simulink model "LandL"  (R2018a)
settings: Solver=VariableStepAuto  StartTime=0.0  StopTime=100  FixedStep=0.0001  MaxStep=1e-2  RelTol=1e-3  EnableMultiTasking=on
values from neighbouring files (symbols this model uses):
  C = (y_hat-y_ref)'*(y_hat-y_ref)/length(y_hat)    [QELandL.m]    (also in QEPID.m)
  ks = K(4)    [QELandL.m]    (also in final_cube_alg.m = x(4))
  pi1 = K(2)*1i    [QELandL.m]    (also in final_cube_alg.m = x(2)*1i)
  pr1 = K(1)    [QELandL.m]    (also in final_cube_alg.m = x(1))
  zr = K(3)    [QELandL.m]    (also in final_cube_alg.m = x(3))
undefined symbols (not defined in the file or in its folder): A, B
libraries: simulink x3, slident x2, cstblocks x1
settings Model: Creator=rromano  LastModifiedBy=Marcelo
settings SolverCC: ZeroCrossAlgorithm=Adaptive  AutoInsertRateTranBlk=on
settings DataIOCC: LimitDataPoints=on  SaveFormat=Array  SignalLoggingSaveFormat=ModelDataLogs
settings OptimizationCC: ExpressionDepthLimit=2147483647  LifeSpan=inf
settings DebuggingCC: AlgebraicLoopMsg=none  UnderspecifiedInitializationDetection=Classic  MergeDetectMultiDrivingBlocksExec=none  MaxConsecutiveZCsMsg=none  SolverPrmCheckMsg=warning  FcnCallInpInsideContextMsg=warning  StateNameClashWarn=warning  SFUnexpectedBacktrackingDiag=warning  SFNoUnconditionalDefaultTransitionDiag=warning  SFExecutionAtInitializationDiag=none
settings HardwareCC: ProdBitPerPointer=32  ProdBitPerSizeT=32  ProdBitPerPtrDiffT=32  ProdLargestAtomicFloat=None  ProdIntDivRoundTo=Undefined  ProdEndianess=Unspecified  ProdWordSize=32  ProdHWDeviceType=32-bit Generic
settings ModelReferenceCC: PropagateSignalLabelsOutOfModel=off
settings CodeAppCC: StateflowObjectComments=on
settings GRTTargetCC: TargetLangStandard=C89/C90 (ANSI)  GeneratePreprocessorConditionals=Disable all  CombineOutputUpdateFcns=off  GRTInterface=on
settings ConfigComp: CovMetricSettings=dw  CovHtmlReporting=on  CovSaveCumulativeToWorkspaceVar=on  CovSaveSingleToWorkspaceVar=on  CovExternalEMLEnable=off

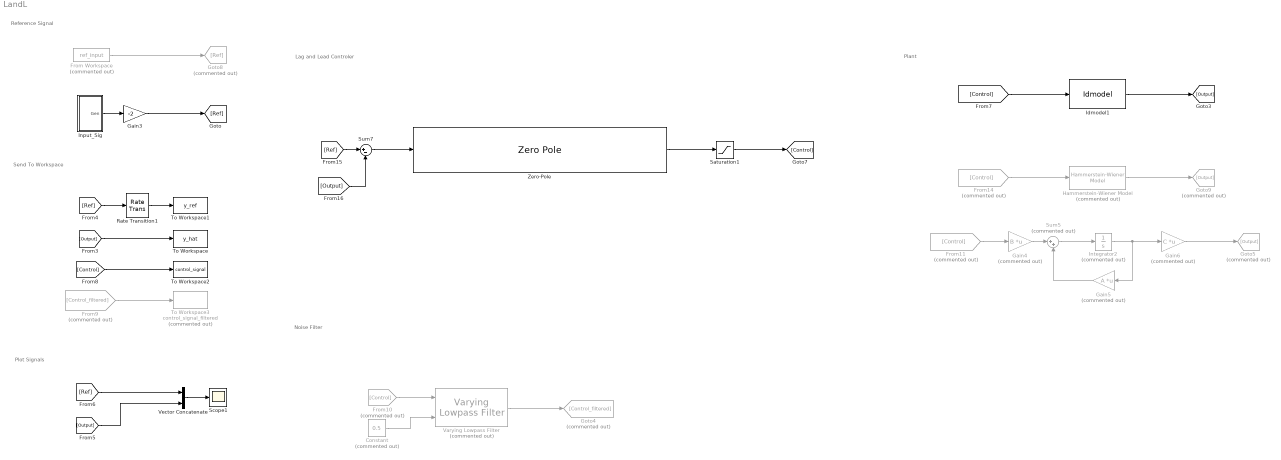
== system LandL ==
  note: Noise Filter
  note: Plot Signals
  note: Send To Workspace
  note: Reference Signal
  note: Lag and Lead Controler
  note: Plant
  Constant : Constant  Commented=on  Value=0.5
  From Workspace : FromWorkspace  Commented=on  VariableName=ref_input  SampleTime=0
  From10 : From  Commented=on  GotoTag=Control
  From11 : From  Commented=on  GotoTag=Control
  From14 : From  Commented=on  GotoTag=Control
  From9 : From  Commented=on  GotoTag=Control_filtered
  Gain3 : Gain  Gain=-2
  Gain4 : Gain  Commented=on  Gain=B  Multiplication=Matrix(K*u)
  Gain5 : Gain  Commented=on  Gain=A  Multiplication=Matrix(K*u)
  Gain6 : Gain  Commented=on  Gain=C  Multiplication=Matrix(K*u)
  Goto4 : Goto  Commented=on  GotoTag=Control_filtered
  Goto5 : Goto  Commented=on  GotoTag=Output
  Goto8 : Goto  Commented=on  GotoTag=Ref
  Goto9 : Goto  Commented=on  GotoTag=Output
  Hammerstein-Wiener Model : slident/Models/Hammerstein-Wiener Model  Commented=on  sys=linear_app  IC=Zero  X0i=0
      settings: SourceProductName=System Identification Toolbox  SourceProductBaseCode=ID
  Idmodel1 : slident/Models/Idmodel  sys=linear_app  IC=0  noi=off  seed=[]
      settings: SourceProductName=System Identification Toolbox  SourceProductBaseCode=ID
  Input_Sig : Subsystem
  Integrator2 : Integrator  Commented=on  ZeroCross=off
  Rate Transition1 : RateTransition  OutPortSampleTime=0.2
  Saturation1 : Saturate  UpperLimit=5000  LowerLimit=-5000
  Scope1 : Scope
  Sum5 : Sum  Commented=on  Inputs=|++
  Sum7 : Sum  Inputs=|+-
  To Workspace : ToWorkspace  VariableName=y_hat  SampleTime=-1
      settings: Save2DSignal=2-D array (concatenate along first dimension)
  To Workspace1 : ToWorkspace  VariableName=y_ref  SampleTime=-1
      settings: Save2DSignal=2-D array (concatenate along first dimension)
  To Workspace2 : ToWorkspace  VariableName=control_signal  SampleTime=-1
      settings: Save2DSignal=2-D array (concatenate along first dimension)
  To Workspace3 : ToWorkspace  Commented=on  VariableName=control_signal_filtered  SaveFormat=Timeseries  SampleTime=-1
      settings: Save2DSignal=2-D array (concatenate along first dimension)
  Varying Lowpass Filter : cstblocks/Linear Parameter Varying/Varying Lowpass Filter  Commented=on  N=1
      settings: SourceProductName=Control System Toolbox
  Vector Concatenate : Concatenate
  Zero-Pole : ZeroPole  Zeros=[-zr]  Poles=[0 -pr1+pi1 -pr1-pi1]  Gain=[ks]
  wires:
  Vector Concatenate/1 -> Scope1/1
  Input_Sig/1(Gen) -> Gain3/1
  [Output] -> To Workspace/1
  [Ref] -> Rate Transition1/1
  [Ref] -> Vector Concatenate/1
  [Output] -> Vector Concatenate/2
  Idmodel1/1 -> [Output]
  [Control] -> Idmodel1/1
  [Control] -> To Workspace2/1
  From9/1 -> To Workspace3/1
  From10/1 -> Varying Lowpass Filter/1
  Constant/1 -> Varying Lowpass Filter/2
  Varying Lowpass Filter/1 -> Goto4/1
  Gain6/1 -> Goto5/1
  From11/1 -> Gain4/1
  Gain4/1 -> Sum5/1
  Sum5/1 -> Integrator2/1
  Gain5/1 -> Sum5/2
  Integrator2/1 -> Gain5/1, Gain6/1
  [Ref] -> Sum7/1
  [Output] -> Sum7/2
  Sum7/1 -> Zero-Pole/1
  Zero-Pole/1 -> Saturation1/1
  Rate Transition1/1 -> To Workspace1/1
  From Workspace/1 -> Goto8/1
  Saturation1/1 -> [Control]
  Hammerstein-Wiener Model/1 -> Goto9/1
  From14/1 -> Hammerstein-Wiener Model/1
  Gain3/1 -> [Ref]

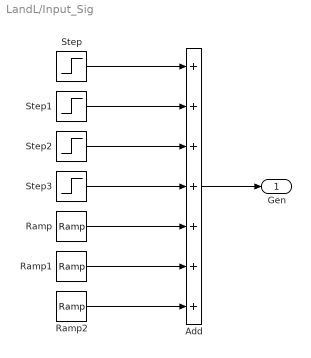
== system LandL/Input_Sig ==
  Add : Sum  Inputs=+++++++
  Ramp : simulink/Sources/Ramp  slope=2  start=70  InitialOutput=0
  Ramp1 : simulink/Sources/Ramp  slope=-4  start=80  InitialOutput=0
  Ramp2 : simulink/Sources/Ramp  slope=2  start=90  InitialOutput=0
  Step : Step  Time=5  After=10  SampleTime=0
  Step1 : Step  Time=25  After=-20  SampleTime=0
  Step2 : Step  Time=35  After=35  SampleTime=0
  Step3 : Step  Time=50  After=-25  SampleTime=0
  Gen : Outport
  wires:
  Ramp1/1 -> Add/6
  Ramp2/1 -> Add/7
  Step3/1 -> Add/4
  Step2/1 -> Add/3
  Ramp/1 -> Add/5
  Add/1 -> Gen/1
  Step1/1 -> Add/2
  Step/1 -> Add/1
